simulink model "turbine_constant_Wt"  (R2016a)
settings: Solver=VariableStepAuto  StartTime=0.0  StopTime=10.0  RelTol=1e-3
undefined symbols (not defined in the file): A, B, D, R, Vw, Wt
settings Model: Creator=hi  LastModifiedBy=hi

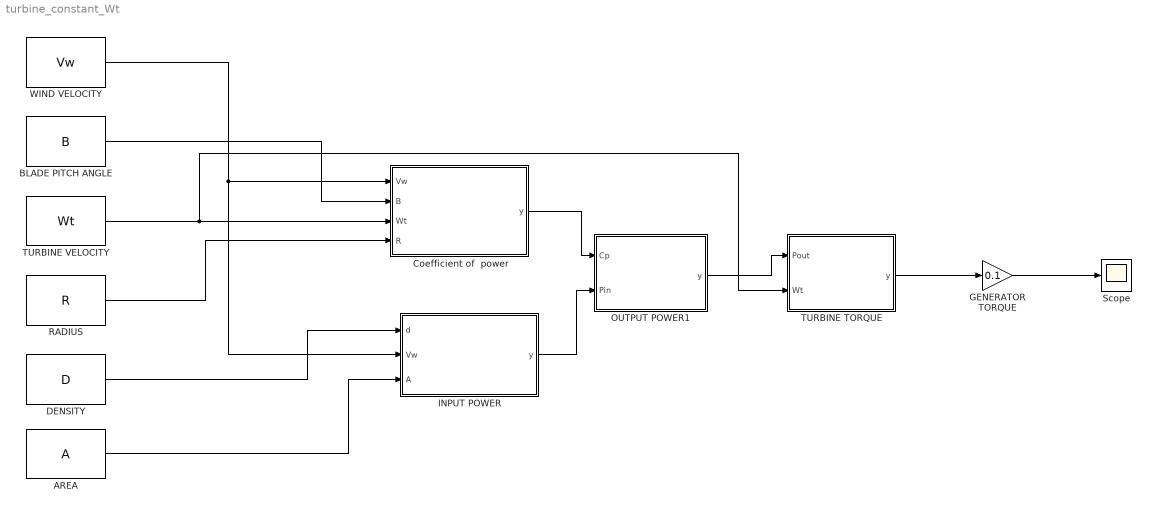
== system turbine_constant_Wt ==
  AREA : Constant  Value=A
  BLADE PITCH ANGLE : Constant  Value=B
  Coefficient of  power : MATLAB Function  TreatAsAtomicUnit=on
  DENSITY : Constant  Value=D
  GENERATOR TORQUE : Gain  Gain=0.1
  INPUT POWER : MATLAB Function  TreatAsAtomicUnit=on
  OUTPUT POWER1 : MATLAB Function  TreatAsAtomicUnit=on
  RADIUS : Constant  Value=R
  Scope : Scope
  TURBINE TORQUE : MATLAB Function  TreatAsAtomicUnit=on
  TURBINE VELOCITY : Constant  Value=Wt
  WIND VELOCITY : Constant  Value=Vw
  wires:
  RADIUS/1 -> Coefficient of  power/4(R)
  BLADE PITCH ANGLE/1 -> Coefficient of  power/2(B)
  WIND VELOCITY/1 -> INPUT POWER/2(Vw), Coefficient of  power/1(Vw)
  DENSITY/1 -> INPUT POWER/1(d)
  AREA/1 -> INPUT POWER/3(A)
  INPUT POWER/1(y) -> OUTPUT POWER1/2(Pin)
  Coefficient of  power/1(y) -> OUTPUT POWER1/1(Cp)
  OUTPUT POWER1/1(y) -> TURBINE TORQUE/1(Pout)
  TURBINE VELOCITY/1 -> TURBINE TORQUE/2(Wt), Coefficient of  power/3(Wt)
  TURBINE TORQUE/1(y) -> GENERATOR TORQUE/1
  GENERATOR TORQUE/1 -> Scope/1

== matlab function turbine_constant_Wt/OUTPUT POWER1 ==
  data: Cp input; y output; Pin input
function y = fcn(Cp,Pin)
%#codegen

y = Cp*Pin;

== matlab function turbine_constant_Wt/INPUT POWER ==
  data: d input; y output; Vw input; A input
function y = fcn(d,Vw,A)
%#codegen

y = 0.5*d*Vw*Vw*Vw*A;

== matlab function turbine_constant_Wt/TURBINE TORQUE ==
  data: Pout input; y output; Wt input
function y = fcn(Pout,Wt)
%#codegen

y = Pout/Wt;

== matlab function turbine_constant_Wt/Coefficient of  power ==
  data: Vw input; y output; B input; Wt input; R input
function y = fcn(Vw,B,Wt,R)
%#codegen
lambda=(Wt*R)/Vw;
ki= (1/(lambda+0.08*B))-(0.035/(B*B*B+1));
y =( 0.5176*(116*ki-0.4*B-5)*exp(-21*ki))+(0.0068*lambda);
